simulink model "BDA_ex1"  (R2023b)
settings: Solver=VariableStepAuto  StartTime=0.0  StopTime=20.0  RelTol=1e-3
values from neighbouring files (symbols this model uses):
  G1_den = [1 2]    [BDA.m]
  G1_num = [1 0]    [BDA.m]
  G2_den = [1 -1]    [BDA.m]
  G2_num = [3 6]    [BDA.m]
  H_den = [1 -2]    [BDA.m]
  H_num = [1 2]    [BDA.m]
settings Model: Creator=Lenovo  LastModifiedBy=Lenovo

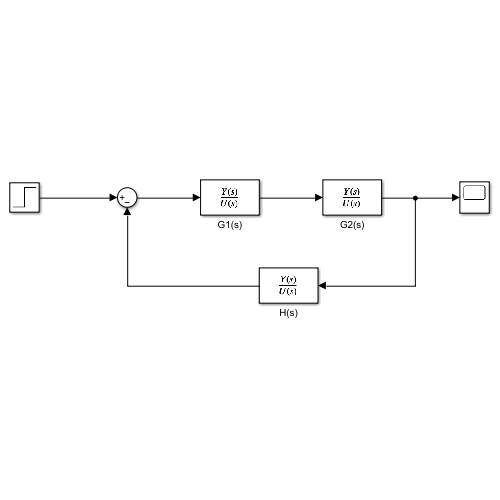
[thumbnail: Simulink's stored preview of the top-level diagram]
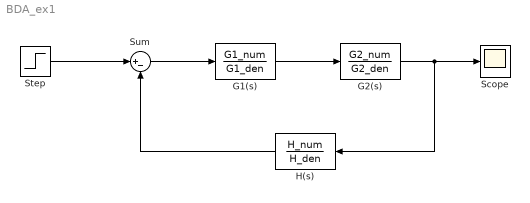
== system BDA_ex1 ==
  G1(s) : TransferFcn  Numerator=G1_num  Denominator=G1_den
  G2(s) : TransferFcn  Numerator=G2_num  Denominator=G2_den
  H(s) : TransferFcn  Numerator=H_num  Denominator=H_den
  Scope : Scope
  Step : Step  Time=0  SampleTime=0
  Sum : Sum  Inputs=|+-
  wires:
  Step/1 -> Sum/1
  Sum/1 -> G1(s)/1
  G1(s)/1 -> G2(s)/1
  G2(s)/1 -> H(s)/1, Scope/1
  H(s)/1 -> Sum/2
